simulink model "Rectifier_Buck_N"  (R2020b)
settings: Solver=VariableStepAuto  StartTime=0.0  StopTime=0.4  RelTol=1e-3
undefined symbols (not defined in the file or in its folder): Acid, Lead
libraries: powerlib x18, dspstat3 x2, electricdrivelib x1, powerlib_meascontrol x1
settings Model: Creator=Alper  LastModifiedBy=mluser

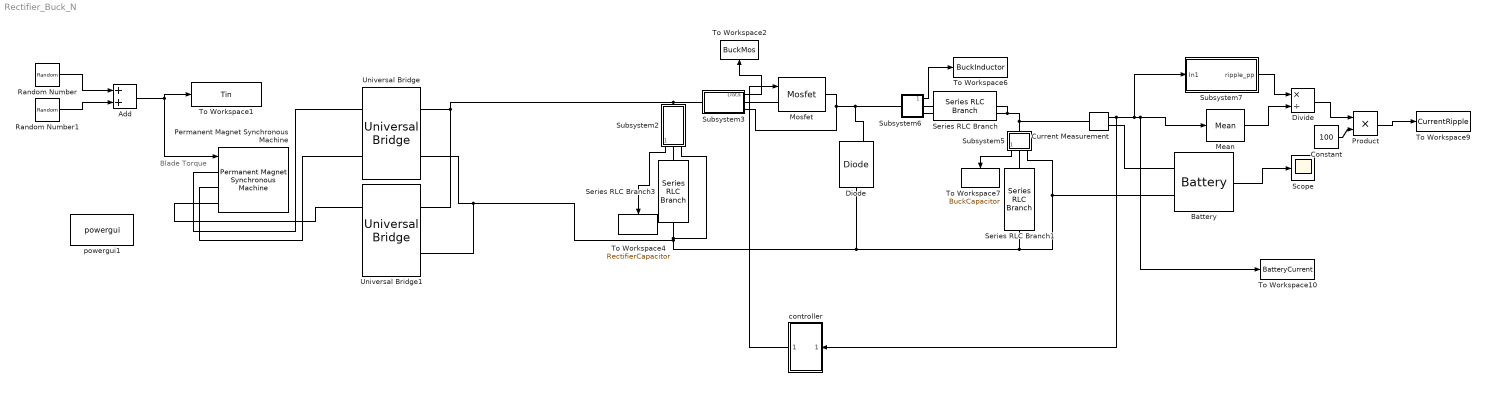
== system Rectifier_Buck_N ==
  note: Blade Torque
  Add : Sum
  Battery : electricdrivelib/Extra Sources/Battery  BatType=Lead-Acid  ShowTempParam=off  ThermalPreset=no  ShowAgeParam=off  NomV=24  NomQ=5.4  SOC=50  Batt_Tr=30  PresetModel=off  MaxQ=5.625  MinV=18  FullV=26.1316  Dis_rate=1.08  R=0.044444  Normal_OP=1.6755  expZone="[24.4342        0.018]"  current=[6.5 13 32.5]  Units=Time  Tci=20  NomT=20  T2=-30  MaxQ2=4.8  FullV2=7.1  Normal_OP2=5.655  expZone2="[6.58           1]"  Rca=0.6  ti=2000  Dp=0  Neq0=0  Tsim=1e6  Ta1=25  Qeol=5.4*0.9  Reol=0.013333*1.2  Char_age=[2.3478, 3]  Dis_age=[2.3478, 10]  N1=1500  N2=10500  N3=1000  N4=1400  Ta2=45  N5=950
  Constant : Constant  Value=100
  Current Measurement : powerlib/Measurements/Current Measurement  PhasorSimulation=off  OutputType=Complex  PSBequivalent=0
  Diode : powerlib/Power Electronics/Diode  Ron=0.001  Lon=0  Vf=1.4  IC=0  UseSnubber=0  Rs=500  Cs=250e-9  Measurements=on
  Divide : Product  Inputs=*/
  Mean : powerlib_meascontrol/Measurements/Mean  Freq=50  Vinit=0  Ts=0
  Mosfet : powerlib/Power Electronics/Mosfet  Ron=3.4  Lon=0.01  Rd=25  Vfd=0  IC=0  Rs=1e5  Cs=inf  Measurements=off
  Permanent Magnet Synchronous Machine : powerlib/Machines/Permanent Magnet Synchronous Machine  NbPhases=3  FluxDistribution=Sinusoidal  RotorType=Round  MechanicalLoad=Torque Tm  PresetModel=No  ShowDetailedParameters=on  MeasurementBus=off  Resistance=10.58  Inductance=8.5e-3  dqInductances=[8.5e-3,8.5e-3]  La=0.0167  MachineConstant=Voltage Constant (V_peak L-L / krpm)  Flux=0.60646  VoltageCst=110  TorqueCst=0.90969  Flat=120  Mechanical=[0.00027 0.005024 1 0]  PolePairs=4  InitialConditions=[300,0, 0,0]  InitialConditions5ph=[0 0 0 0 0 0]  RefAngle=90 degrees behind phase A axis (modified Park)  IterativeDiscreteModel=Trapezoidal non iterative  TsBlock=-1  TsPowergui=0
  Product : Product
  Random Number : RandomNumber  Mean=-1.6  Variance=0.05  SampleTime=1
  Random Number1 : RandomNumber  Variance=0.1  SampleTime=1e-3
  Scope : Scope
  Series RLC Branch : powerlib/Elements/Series RLC Branch  LConnTagsString=__new0  RConnTagsString=__new0  BranchType=RL  Resistance=0.07  Inductance=2.2e-3  SetiL0=off  InitialCurrent=0  Capacitance=1e-6  Setx0=off  InitialVoltage=0  Measurements=None
  Series RLC Branch1 : powerlib/Elements/Series RLC Branch  LConnTagsString=__new0  RConnTagsString=__new0  BranchType=RC  Resistance=0.360  Inductance=1e-3  SetiL0=off  InitialCurrent=0  Capacitance=20e-6  Setx0=off  InitialVoltage=0  Measurements=None
  Series RLC Branch3 : powerlib/Elements/Series RLC Branch  LConnTagsString=__new0  RConnTagsString=__new0  BranchType=C  Resistance=1  Inductance=1e-3  SetiL0=off  InitialCurrent=0  Capacitance=220e-6  Setx0=on  InitialVoltage=300  Measurements=None
  Subsystem2 : Subsystem
  Subsystem3 : Subsystem
  Subsystem5 : Subsystem
  Subsystem6 : Subsystem
  Subsystem7 : Subsystem
  To Workspace1 : ToWorkspace  VariableName=Tin  SaveFormat=Timeseries  SampleTime=-1
  To Workspace10 : ToWorkspace  VariableName=BatteryCurrent  SaveFormat=Timeseries  SampleTime=-1
  To Workspace2 : ToWorkspace  VariableName=BuckMos  SaveFormat=Timeseries  SampleTime=-1
  To Workspace4 : ToWorkspace  VariableName=RectifierCapacitor  SaveFormat=Timeseries  SampleTime=-1
  To Workspace6 : ToWorkspace  VariableName=BuckInductor  SaveFormat=Timeseries  SampleTime=-1
  To Workspace7 : ToWorkspace  VariableName=BuckCapacitor  SaveFormat=Timeseries  SampleTime=-1
  To Workspace9 : ToWorkspace  VariableName=CurrentRipple  SaveFormat=Timeseries  SampleTime=-1
  Universal Bridge : powerlib/Power Electronics/Universal Bridge  Arms=2  SnubberResistance=1e5  SnubberCapacitance=inf  Device=Diodes  Ron=1e-3  Lon=0  ForwardVoltages="[  0  0  ]"  ForwardVoltage=0.9  GTOparameters=[ 10e-6 , 20e-6 ]  IGBTparameters=[ 1e-6 , 2e-6 ]  Measurements=None  Measurements_2=None  converterType=Rectifier
  Universal Bridge1 : powerlib/Power Electronics/Universal Bridge  Arms=2  SnubberResistance=1e5  SnubberCapacitance=inf  Device=Diodes  Ron=1e-3  Lon=0  ForwardVoltages="[  0  0  ]"  ForwardVoltage=0.9  GTOparameters=[ 10e-6 , 20e-6 ]  IGBTparameters=[ 1e-6 , 2e-6 ]  Measurements=None  Measurements_2=None  converterType=Rectifier
  controller : Subsystem
  powergui1 : powerlib/powergui  Priority=1  SimulationMode=Discrete  SampleTime=1e-6  frequency=60  Iterations=50  frequencyindice=0  Pbase=100e6  ErrMax=1e-4  UnitsV=kV  UnitsW=MW  buscounter=0  FunctionMessages=off  echomessages=off  EnableUseOfTLC=off  CurrentSourceSwitches=off  DisableSnubberDevices=off  DisableRonSwitches=off  DisableVfSwitches=off  DisplayEquations=off  AutomaticDiscreteSolvers=off  SolverType=Tustin/Backward Euler (TBE)  Interpol=off  ExternalGateDelay=off  methode=off  Ts=100  x0status=blocks  SPID=on  SwTol=0  HookPort=off  NonlinearTolerance=0  nMaxIteration=15  ContinueOnMaxIteration=off  RestoreLinks=warning  ResistiveCurrentMeasurement=off  Frange=[0:2:500]  Ylog=off  Xlog=on  ShowGrid=off  save=off  variable=ZData  structure=0  ZoomFFT=off  StartTime=0.0  cycles=1  DisplayStyle=1  fundamental=60  FreqAxis=off  MaxFrequency=1000  frequencyindicesteady=1  RmsSteady=1  display=off
  wires:
  Random Number1/1 -> Add/2
  Random Number/1 -> Add/1
  Battery/1 -> Scope/1
  Current Measurement/1 -> Subsystem7/1(In1), To Workspace10/1, Mean/1, controller/1(In1)
  Subsystem2/1(Data) -> To Workspace4/1
  Subsystem3/1(Data) -> To Workspace2/1
  Subsystem6/1(Data) -> To Workspace6/1
  Subsystem5/1(Data) -> To Workspace7/1
  controller/1(Out1) -> Mosfet/1
  Mean/1 -> Divide/2
  Subsystem7/1(ripple_pp) -> Divide/1
  Divide/1 -> Product/1
  Constant/1 -> Product/2
  Product/1 -> To Workspace9/1
  Add/1 -> To Workspace1/1, Permanent Magnet Synchronous Machine/1
  connections:
  Permanent Magnet Synchronous Machine/LConn1 -- Universal Bridge/LConn1
  Universal Bridge1/LConn1 -- Permanent Magnet Synchronous Machine/LConn3
  Permanent Magnet Synchronous Machine/LConn2 -- Universal Bridge/LConn2
  Series RLC Branch3/LConn1 -- Subsystem2/RConn1
  Universal Bridge1/RConn1 -- Subsystem3/LConn1 -- Subsystem2/LConn1 -- Universal Bridge/RConn1
  Subsystem3/RConn1 -- Mosfet/LConn1
  Subsystem2/RConn2 -- Series RLC Branch3/RConn1 -- Universal Bridge1/RConn2 -- Universal Bridge/RConn2 -- Diode/LConn1 -- Battery/LConn2 -- Subsystem5/RConn2 -- Series RLC Branch1/RConn1
  Subsystem3/RConn2 -- Diode/RConn1 -- Subsystem6/LConn1 -- Mosfet/RConn1
  Series RLC Branch1/LConn1 -- Subsystem5/RConn1
  Subsystem6/RConn1 -- Series RLC Branch/LConn1
  Subsystem6/RConn2 -- Current Measurement/LConn1 -- Subsystem5/LConn1 -- Series RLC Branch/RConn1
  Current Measurement/RConn1 -- Battery/LConn1

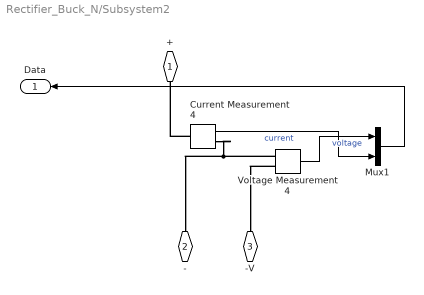
== system Rectifier_Buck_N/Subsystem2 ==
  Current Measurement4 : powerlib/Measurements/Current Measurement  PhasorSimulation=off  OutputType=Complex  PSBequivalent=0
  Mux1 : Mux  Inputs=2
  Voltage Measurement4 : powerlib/Measurements/Voltage Measurement  PhasorSimulation=off  OutputType=Complex  PSBequivalent=0
  + : PMIOPort  Side=Left
  - : PMIOPort  Port=2  Side=Right
  -V : PMIOPort  Port=3  Side=Right
  Data : Outport
  wires:
  Mux1/1 -> Data/1
  Voltage Measurement4/1 -> Mux1/1  "voltage"
  Current Measurement4/1 -> Mux1/2  "current"
  connections:
  Voltage Measurement4/LConn2 -- -V/RConn1
  Current Measurement4/LConn1 -- +/RConn1
  Current Measurement4/RConn1 -- Voltage Measurement4/LConn1 -- -/RConn1

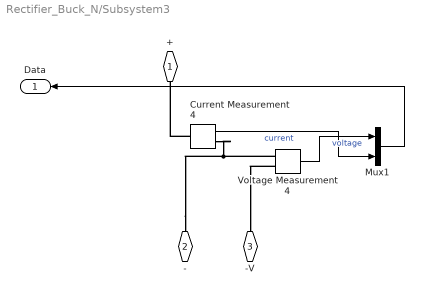
== system Rectifier_Buck_N/Subsystem3 ==
  Current Measurement4 : powerlib/Measurements/Current Measurement  PhasorSimulation=off  OutputType=Complex  PSBequivalent=0
  Mux1 : Mux  Inputs=2
  Voltage Measurement4 : powerlib/Measurements/Voltage Measurement  PhasorSimulation=off  OutputType=Complex  PSBequivalent=0
  + : PMIOPort  Side=Left
  - : PMIOPort  Port=2  Side=Right
  -V : PMIOPort  Port=3  Side=Right
  Data : Outport
  wires:
  Current Measurement4/1 -> Mux1/2  "current"
  Voltage Measurement4/1 -> Mux1/1  "voltage"
  Mux1/1 -> Data/1
  connections:
  -/RConn1 -- Voltage Measurement4/LConn1 -- Current Measurement4/RConn1
  Current Measurement4/LConn1 -- +/RConn1
  Voltage Measurement4/LConn2 -- -V/RConn1

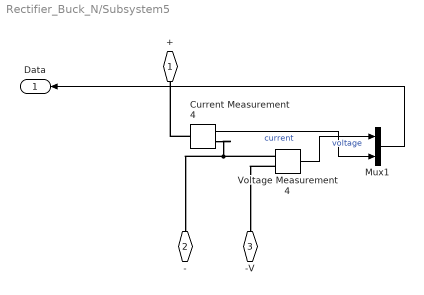
== system Rectifier_Buck_N/Subsystem5 ==
  Current Measurement4 : powerlib/Measurements/Current Measurement  PhasorSimulation=off  OutputType=Complex  PSBequivalent=0
  Mux1 : Mux  Inputs=2
  Voltage Measurement4 : powerlib/Measurements/Voltage Measurement  PhasorSimulation=off  OutputType=Complex  PSBequivalent=0
  + : PMIOPort  Side=Left
  - : PMIOPort  Port=2  Side=Right
  -V : PMIOPort  Port=3  Side=Right
  Data : Outport
  wires:
  Mux1/1 -> Data/1
  Voltage Measurement4/1 -> Mux1/1  "voltage"
  Current Measurement4/1 -> Mux1/2  "current"
  connections:
  Voltage Measurement4/LConn2 -- -V/RConn1
  Current Measurement4/LConn1 -- +/RConn1
  Current Measurement4/RConn1 -- Voltage Measurement4/LConn1 -- -/RConn1

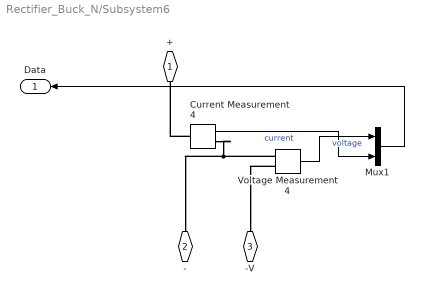
== system Rectifier_Buck_N/Subsystem6 ==
  Current Measurement4 : powerlib/Measurements/Current Measurement  PhasorSimulation=off  OutputType=Complex  PSBequivalent=0
  Mux1 : Mux  Inputs=2
  Voltage Measurement4 : powerlib/Measurements/Voltage Measurement  PhasorSimulation=off  OutputType=Complex  PSBequivalent=0
  + : PMIOPort  Side=Left
  - : PMIOPort  Port=2  Side=Right
  -V : PMIOPort  Port=3  Side=Right
  Data : Outport
  wires:
  Mux1/1 -> Data/1
  Voltage Measurement4/1 -> Mux1/1  "voltage"
  Current Measurement4/1 -> Mux1/2  "current"
  connections:
  Voltage Measurement4/LConn2 -- -V/RConn1
  Current Measurement4/LConn1 -- +/RConn1
  Current Measurement4/RConn1 -- Voltage Measurement4/LConn1 -- -/RConn1

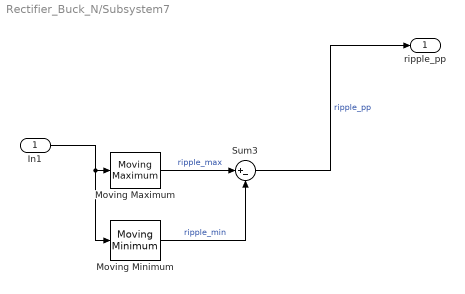
== system Rectifier_Buck_N/Subsystem7 ==
  In1 : Inport
  Moving Maximum : dspstat3/Moving Maximum  SpecifyWindowLength=on  WindowLength=5e3  SimulateUsing=Code generation
      settings: SourceProductBaseCode=DS
  Moving Minimum : dspstat3/Moving Minimum  SpecifyWindowLength=on  WindowLength=5e3  SimulateUsing=Code generation
      settings: SourceProductBaseCode=DS
  Sum3 : Sum  Inputs=|+-
  ripple_pp : Outport
  wires:
  Moving Minimum/1 -> Sum3/2  "ripple_min"
  In1/1 -> Moving Minimum/1, Moving Maximum/1
  Moving Maximum/1 -> Sum3/1  "ripple_max"
  Sum3/1 -> ripple_pp/1  "ripple_pp"

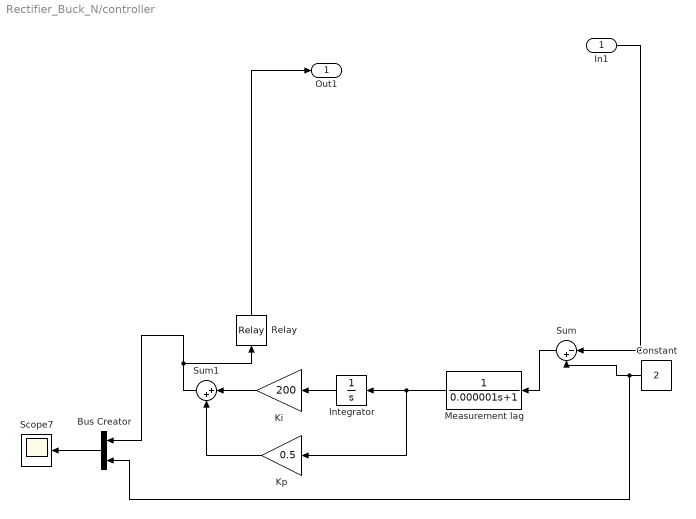
== system Rectifier_Buck_N/controller ==
  In1 : Inport
  Bus Creator : BusCreator  Inputs=2
  Constant : Constant  Value=2
  Integrator : Integrator
  Ki : Gain  Gain=200
  Kp : Gain  Gain=0.5
  Measurement lag : TransferFcn  Denominator=[0.000001 1]
  Relay : Relay
  Scope7 : Scope
  Sum : Sum  Inputs=|-+  InputSameDT=on  SaturateOnIntegerOverflow=on  OutDataTypeStr=Inherit: Same as first input
  Sum1 : Sum  Inputs=|++  InputSameDT=on  SaturateOnIntegerOverflow=on  OutDataTypeStr=Inherit: Same as first input
  Out1 : Outport
  wires:
  Integrator/1 -> Ki/1
  In1/1 -> Sum/1
  Constant/1 -> Bus Creator/2, Sum/2
  Kp/1 -> Sum1/2
  Bus Creator/1 -> Scope7/1
  Sum1/1 -> Bus Creator/1, Relay/1
  Sum/1 -> Measurement lag/1
  Relay/1 -> Out1/1
  Ki/1 -> Sum1/1
  Measurement lag/1 -> Integrator/1, Kp/1
